simulink model "stateflowdemo"  (R2020b)
settings: Solver=VariableStepAuto  StartTime=0.0  StopTime=10.0  RelTol=1e-3
settings Model: Creator=Training  LastModifiedBy=Training

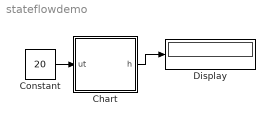
== system stateflowdemo ==
  Chart : Stateflow chart  TreatAsAtomicUnit=on
  Constant : Constant  Value=20
  Display : Display
  wires:
  Chart/1(h) -> Display/1
  Constant/1 -> Chart/1(ut)

== stateflow chart stateflowdemo/Chart ==
  (default) -> (junction 11) : {at=23;}
  (junction 11) -> (junction 12) [order 1] : [at>ut]
  (junction 11) -> (junction 13) [order 2]
  (junction 12) -> (junction 17) : {h = -1;}
  (junction 13) -> (junction 14) [order 1] : [at<ut]
  (junction 13) -> (junction 15) [order 2] : {h = 0;}
  (junction 14) -> (junction 16) : {h = 1;}
  (junction 16) -> (junction 15)
  (junction 17) -> (junction 16)
  (junction 15) -> (junction 18)
  data: at local; h output; ut input
